simulink model "PerturbedCartesianOrbitPropagatorDV"  (R2023a)
settings: Solver=ode4  StartTime=0.0  StopTime=10.0  FixedStep=dt  MaxStep=max_step_size  RelTol=relative_tolerance
settings Model: Creator=ndelurgio  LastModifiedBy=ndelurgio

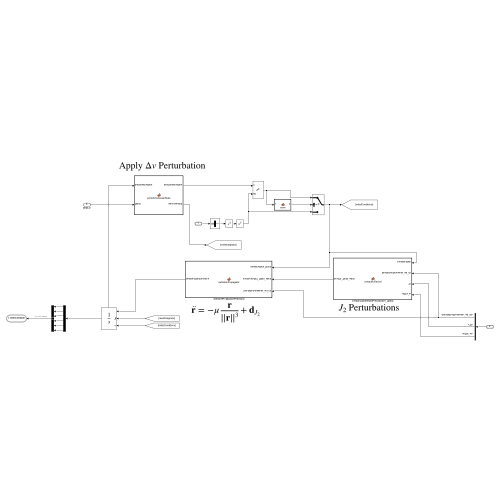
[thumbnail: Simulink's stored preview of the top-level diagram]
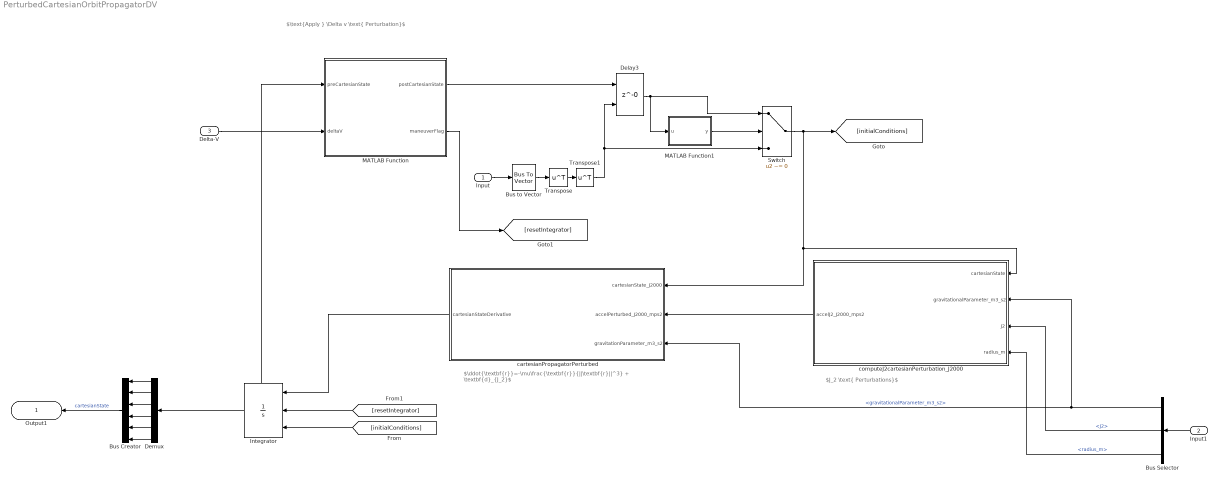
== system PerturbedCartesianOrbitPropagatorDV ==
  note: $J_2 \text{ Perturbations}$
  note: $\ddot{\textbf{r}}=-\mu\frac{\textbf{r}}{||\textbf{r}||^3} + \textbf{d}_{J_2}$
  note: $\text{Apply } \Delta v \text{ Perturbation}$
  Input : Inport  OutDataTypeStr=Bus: cartesianState
  Input1 : Inport  Port=2  OutDataTypeStr=Bus: earthProperties
  Delta-V : Inport  Port=3  PortDimensions=3
  Bus Creator : BusCreator  Inputs=6  OutDataTypeStr=Bus: cartesianState  NonVirtualBus=on
      settings: InheritFromInputs=off
  Bus Selector : BusSelector  OutputSignals=gravitationalParameter_m3_s2,J2,radius_m
  Bus to Vector : BusToVector
  Delay3 : Delay  DelayLength=0  InitialConditionSource=Input port  InitialCondition=[0,0,0,0,0,0]
      settings: InputPortMap=u0,p4
  Demux : Demux  Outputs=6
  Integrator : Integrator  ExternalReset=rising  InitialConditionSource=external  ShowStatePort=on
  MATLAB Function : MATLAB Function  TreatAsAtomicUnit=on
  MATLAB Function1 : MATLAB Function  TreatAsAtomicUnit=on
  Switch : Switch  Criteria=u2 ~= 0  SaturateOnIntegerOverflow=off  InputSameDT=off
  Transpose : Math  Operator=transpose
  Transpose1 : Math  Operator=transpose
  cartesianPropagatorPerturbed : MATLAB Function  TreatAsAtomicUnit=on
  computeJ2cartesianPerturbation_J2000 : MATLAB Function  TreatAsAtomicUnit=on
  Output1 : Outport  OutDataTypeStr=Bus: cartesianState
  wires:
  Input/1 -> Bus to Vector/1
  Bus to Vector/1 -> Transpose/1
  computeJ2cartesianPerturbation_J2000/1(accelJ2_J2000_mps2) -> cartesianPropagatorPerturbed/2(accelPerturbed_J2000_mps2)
  Input1/1 -> Bus Selector/1
  Bus Selector/1 -> cartesianPropagatorPerturbed/3(gravitationParameter_m3_s2), computeJ2cartesianPerturbation_J2000/2(gravitationalParameter_m3_s2)  "<gravitationalParameter_m3_s2>"
  Bus Selector/2 -> computeJ2cartesianPerturbation_J2000/3(J2)  "<J2>"
  Bus Selector/3 -> computeJ2cartesianPerturbation_J2000/4(radius_m)  "<radius_m>"
  Demux/2 -> Bus Creator/2
  Bus Creator/1 -> Output1/1  "cartesianState"
  Demux/3 -> Bus Creator/3
  Demux/1 -> Bus Creator/1
  Demux/6 -> Bus Creator/6
  Demux/5 -> Bus Creator/5
  Demux/4 -> Bus Creator/4
  Delta-V/1 -> MATLAB Function/2(deltaV)
  [initialConditions] -> Integrator/3
  [resetIntegrator] -> Integrator/2
  MATLAB Function/2(maneuverFlag) -> [resetIntegrator]
  MATLAB Function/1(postCartesianState) -> Delay3/1
  Integrator/State -> MATLAB Function/1(preCartesianState)
  cartesianPropagatorPerturbed/1(cartesianStateDerivative) -> Integrator/1
  Delay3/1 -> Switch/1, MATLAB Function1/1(u)
  Switch/1 -> computeJ2cartesianPerturbation_J2000/1(cartesianState), cartesianPropagatorPerturbed/1(cartesianState_J2000), [initialConditions]
  MATLAB Function1/1(y) -> Switch/2
  Transpose1/1 -> Switch/3, Delay3/2
  Transpose/1 -> Transpose1/1
  Integrator/1 -> Demux/1

== matlab function PerturbedCartesianOrbitPropagatorDV/cartesianPropagatorPerturbed ==
  data: cartesianState_J2000 input; cartesianStateDerivative output; accelPerturbed_J2000_mps2 input; gravitationParameter_m3_s2 input
function cartesianStateDerivative = cartesianPropagator(cartesianState_J2000,accelPerturbed_J2000_mps2,gravitationParameter_m3_s2)

cartesianStateDerivative = cartesianPropagatorPerturbed(cartesianState_J2000,accelPerturbed_J2000_mps2,gravitationParameter_m3_s2);

end

== matlab function PerturbedCartesianOrbitPropagatorDV/computeJ2cartesianPerturbation_J2000 ==
  data: cartesianState input; accelJ2_J2000_mps2 output; gravitationalParameter_m3_s2 input; J2 input; radius_m input
function accelJ2_J2000_mps2 = computeJ2accel(cartesianState,gravitationalParameter_m3_s2,J2,radius_m)

accelJ2_J2000_mps2 = computeJ2cartesianPerturbation_J2000(cartesianState,gravitationalParameter_m3_s2,J2,radius_m);

end

== matlab function PerturbedCartesianOrbitPropagatorDV/MATLAB Function ==
  data: preCartesianState input; postCartesianState output; deltaV input; maneuverFlag output
function [postCartesianState,maneuverFlag] = perturbCartesianState(preCartesianState,deltaV)
[postCartesianState,maneuverFlag] = perturbCartesianState(preCartesianState,deltaV);
end

== matlab function PerturbedCartesianOrbitPropagatorDV/MATLAB Function1 ==
  data: u input; y output
function y = norm(u)

y = norm(u);
end
